simulink model "Battery_Thevenin_Model_R"  (R2025a)
settings: Solver=ode1  StartTime=0.0  StopTime=Ttotal  FixedStep=Tsample  MaxStep=1e-3  RelTol=1e-3
values from neighbouring files (symbols this model uses):
  C_init = C_total*.8    (= 259200)    [Battery_Parameters_R.m]
  C_nom = 90    [Battery_Parameters_R.m]
  C_total = C_nom*3600    (= 324000)    [Battery_Parameters_R.m]
  Rbat = (D10A(5,2)-D20A(5,2))/10    [Battery_Parameters_R.m]
  Ttotal = 3600*4    (= 14400)    [Battery_Parameters_R.m]
undefined symbols (not defined in the file or in its folder): P01A
settings Model: Creator=mwxiao  LastModifiedBy=dsh253
settings SolverCC: AlgebraicLoopSolver=TrustRegion
settings DataIOCC: LimitDataPoints=on  SaveFormat=Array  SignalLoggingSaveFormat=ModelDataLogs  ReturnWorkspaceOutputs=off  SignalLoggingName=sigsOut
settings OptimizationCC: ExpressionDepthLimit=2147483647.0  LifeSpan=inf
settings DebuggingCC: SaveWithParameterizedLinksMsg=none  UnderspecifiedInitializationDetection=Classic  MergeDetectMultiDrivingBlocksExec=none  SignalResolutionControl=TryResolveAllWithWarning  MultiTaskDSMMsg=warning  MultiTaskCondExecSysMsg=none  FcnCallInpInsideContextMsg=warning  UnconnectedInputMsg=warning  UnconnectedOutputMsg=warning  UnconnectedLineMsg=warning  StateNameClashWarn=warning  SFUnexpectedBacktrackingDiag=warning  SFNoUnconditionalDefaultTransitionDiag=warning  SFExecutionAtInitializationDiag=none  ArithmeticOperatorsInVariantConditions=warning
settings HardwareCC: ProdBitPerPointer=32.0  ProdBitPerSizeT=32.0  ProdBitPerPtrDiffT=32.0  ProdLargestAtomicFloat=None  ProdIntDivRoundTo=Undefined  ProdEndianess=Unspecified  ProdWordSize=32.0  ProdHWDeviceType=32-bit Generic  TargetUnknown=on
settings ModelReferenceCC: EnableRefExpFcnMdlSchedulingChecks=on  PropagateSignalLabelsOutOfModel=off
settings SFSimCC: SimUseLocalCustomCode=off  CustomCodeUndefinedFunction=UseInterfaceOnly
settings RTWCC: RTWUseLocalCustomCode=off  GPUComputeCapability=3.5  DLArmComputeVersion=19.05
settings CodeAppCC: StateflowObjectComments=on
settings GRTTargetCC: TargetLangStandard=C89/C90 (ANSI)  CombineOutputUpdateFcns=off  GRTInterface=on
settings ConfigComp: CovMetricSettings=dw  CovSaveCumulativeToWorkspaceVar=on  CovSaveSingleToWorkspaceVar=on  CovExternalEMLEnable=off

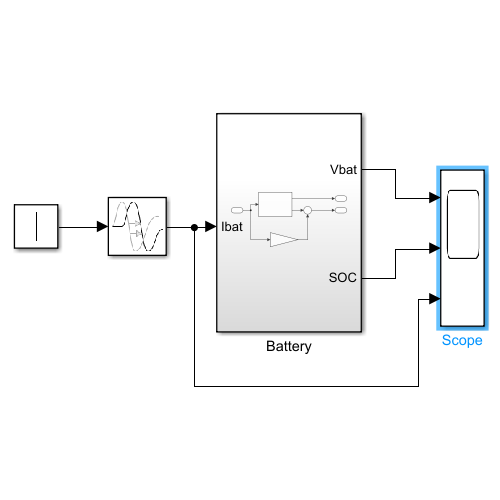
[thumbnail: Simulink's stored preview of the top-level diagram]
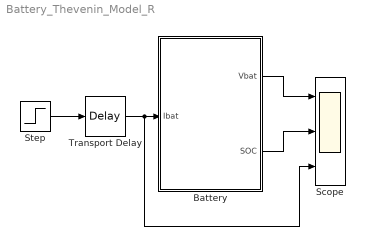
== system Battery_Thevenin_Model_R ==
  Battery : Subsystem
  Scope : Scope  NumInputPorts=3
      settings: ActiveDisplayYMinimum=11.652574070836538  ActiveDisplayYMaximum=13.8564997309695
  Step : Step  Time=(Ttotal/2) - 900  Before=C_nom/3  After=-C_nom/3  SampleTime=0
  Transport Delay : TransportDelay  DelayTime=1200
  wires:
  Transport Delay/1 -> Scope/3, Battery/1(Ibat)
  Step/1 -> Transport Delay/1
  Battery/2(SOC) -> Scope/2
  Battery/1(Vbat) -> Scope/1

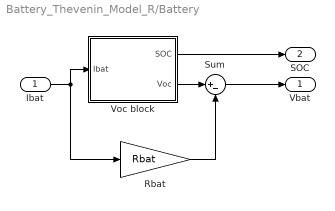
== system Battery_Thevenin_Model_R/Battery ==
  Ibat : Inport
  Rbat : Gain  Gain=Rbat
  Sum : Sum  Inputs=|+-
  Voc block : Subsystem
  Vbat : Outport
  SOC : Outport  Port=2
  wires:
  Ibat/1 -> Rbat/1, Voc block/1(Ibat)
  Rbat/1 -> Sum/2
  Sum/1 -> Vbat/1
  Voc block/2(Voc) -> Sum/1
  Voc block/1(SOC) -> SOC/1

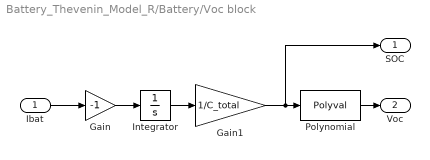
== system Battery_Thevenin_Model_R/Battery/Voc block ==
  Ibat : Inport
  Gain : Gain  Gain=-1
  Gain1 : Gain  Gain=1/C_total
  Integrator : Integrator  InitialCondition=C_init  LimitOutput=on  UpperSaturationLimit=C_total  LowerSaturationLimit=0
  Polynomial : Polyval  Coefs=P01A
  SOC : Outport
  Voc : Outport  Port=2
  wires:
  Gain/1 -> Integrator/1
  Integrator/1 -> Gain1/1
  Ibat/1 -> Gain/1
  Gain1/1 -> SOC/1, Polynomial/1
  Polynomial/1 -> Voc/1
